simulink model "enmod"  (R2021b)
settings: Solver=VariableStepAuto  StartTime=0.0  StopTime=3000  RelTol=1e-3
libraries: dsparch4 x2
settings Model: Creator=lucas  LastModifiedBy=lucas

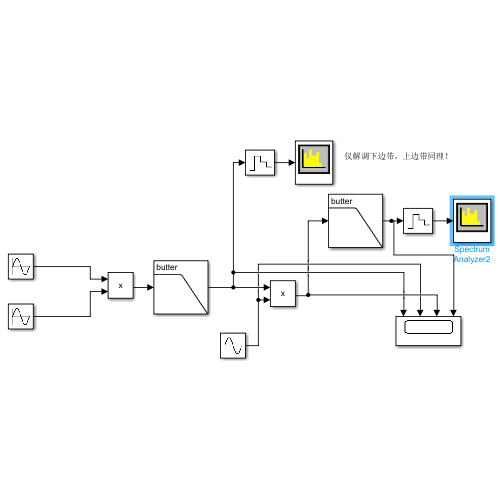
[thumbnail: Simulink's stored preview of the top-level diagram]
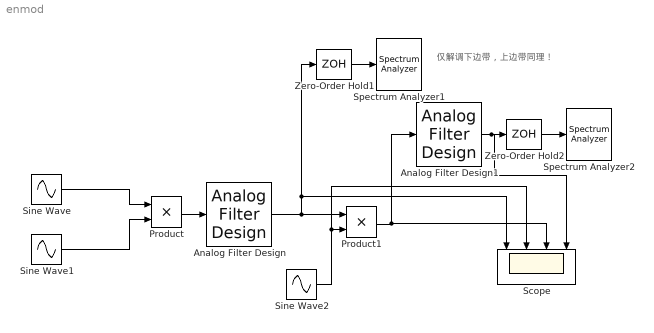
== system enmod ==
  note: 仅解调下边带，上边带同理！
  Analog Filter Design : dsparch4/Analog Filter Design  method=Butterworth  filttype=Lowpass  N=10  Wlo=2*pi*18  Whi=80  Rp=2  Rs=40
  Analog Filter Design1 : dsparch4/Analog Filter Design  method=Butterworth  filttype=Lowpass  N=10  Wlo=2*pi*18  Whi=80  Rp=2  Rs=40
  Product : Product
  Product1 : Product
  Scope : Scope  NumInputPorts=4
  Sine Wave : Sin  Amplitude=2  Frequency=2*pi*2  SampleTime=0
  Sine Wave1 : Sin  Amplitude=2  Frequency=2*pi*20  SampleTime=0
  Sine Wave2 : Sin  Amplitude=2  Frequency=2*pi*20  SampleTime=0
  Spectrum Analyzer1 : SpectrumAnalyzer
  Spectrum Analyzer2 : SpectrumAnalyzer
  Zero-Order Hold1 : ZeroOrderHold  SampleTime=-1
  Zero-Order Hold2 : ZeroOrderHold  SampleTime=-1
  wires:
  Zero-Order Hold2/1 -> Spectrum Analyzer2/1
  Product/1 -> Analog Filter Design/1
  Sine Wave/1 -> Product/1
  Sine Wave1/1 -> Product/2
  Analog Filter Design/1 -> Zero-Order Hold1/1, Scope/1, Product1/1
  Sine Wave2/1 -> Scope/2, Product1/2
  Analog Filter Design1/1 -> Scope/4, Zero-Order Hold2/1
  Product1/1 -> Analog Filter Design1/1, Scope/3
  Zero-Order Hold1/1 -> Spectrum Analyzer1/1
